simulink model "multibus_signal_routing"  (R2021a)
settings: Solver=VariableStepAuto  StartTime=0.0  StopTime=10.0  RelTol=1e-3
libraries: simulink x1
settings Model: Creator=Acer  LastModifiedBy=Acer

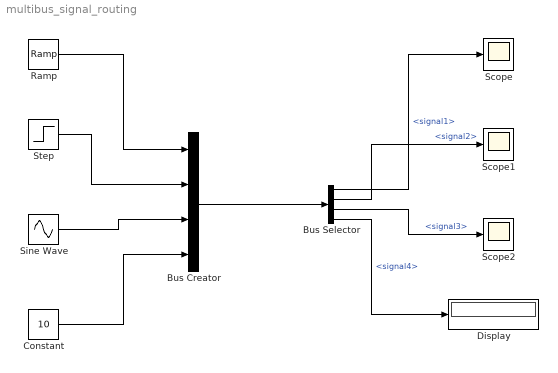
== system multibus_signal_routing ==
  Bus Creator : BusCreator  Inputs=4
  Bus Selector : BusSelector  OutputSignals=signal1,signal2,signal3,signal4
  Constant : Constant  Value=10
  Display : Display
  Ramp : simulink/Sources/Ramp  slope=1  start=0  InitialOutput=0
  Scope : Scope
  Scope1 : Scope
  Scope2 : Scope
  Sine Wave : Sin  SampleTime=0
  Step : Step  SampleTime=0
  wires:
  Ramp/1 -> Bus Creator/1
  Step/1 -> Bus Creator/2
  Sine Wave/1 -> Bus Creator/3
  Constant/1 -> Bus Creator/4
  Bus Creator/1 -> Bus Selector/1
  Bus Selector/1 -> Scope/1  "<signal1>"
  Bus Selector/2 -> Scope1/1  "<signal2>"
  Bus Selector/3 -> Scope2/1  "<signal3>"
  Bus Selector/4 -> Display/1  "<signal4>"
